simulink model "Problem_No3"  (R2020a)
settings: Solver=ode45  StartTime=0.0  StopTime=10.0  MaxStep=0.001  RelTol=1e-3
model workspace (MAT data in the model file):
  h2r = 5
settings Model: Creator='Z'ome  LastModifiedBy=Animesh Uttekar

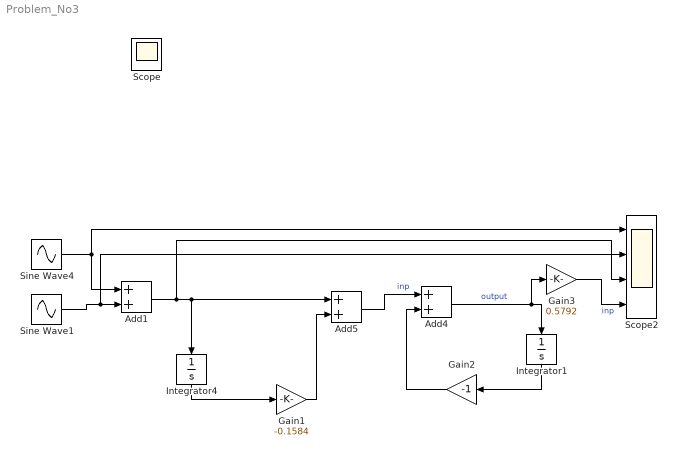
== system Problem_No3 ==
  Add1 : Sum
  Add4 : Sum
  Add5 : Sum
  Gain1 : Gain  Gain=-0.1584
  Gain2 : Gain  Gain=-1
  Gain3 : Gain  Gain=0.5792
  Integrator1 : Integrator
  Integrator4 : Integrator
  Scope2 : Scope  NumInputPorts=4
  Sine Wave1 : Sin  Frequency=100  SampleTime=0
  Sine Wave4 : Sin  SampleTime=0
  Scope : Scope
  wires:
  Sine Wave1/1 -> Add1/2, Scope2/2
  Sine Wave4/1 -> Add1/1, Scope2/1
  Add1/1 -> Add5/1, Integrator4/1, Scope2/3
  Integrator1/1 -> Gain2/1
  Gain2/1 -> Add4/2
  Add4/1 -> Gain3/1, Integrator1/1  "output"
  Add5/1 -> Add4/1  "inp"
  Integrator4/1 -> Gain1/1
  Gain1/1 -> Add5/2
  Gain3/1 -> Scope2/4  "inp"
